simulink model "simulationSprint2"  (R2018b)
settings: Solver=FixedStepAuto  StartTime=0.0  StopTime=10  FixedStep=0.01  MaxStep=100e-3  RelTol=1e-3
(part 1 of 3)
settings Model: Creator=ADEMATO1  LastModifiedBy=afonso
settings SolverCC: PositivePriorityOrder=on  AutoInsertRateTranBlk=on  InsertRTBMode=Always
settings DataIOCC: ReturnWorkspaceOutputs=on
settings DebuggingCC: StringTruncationChecking=warning

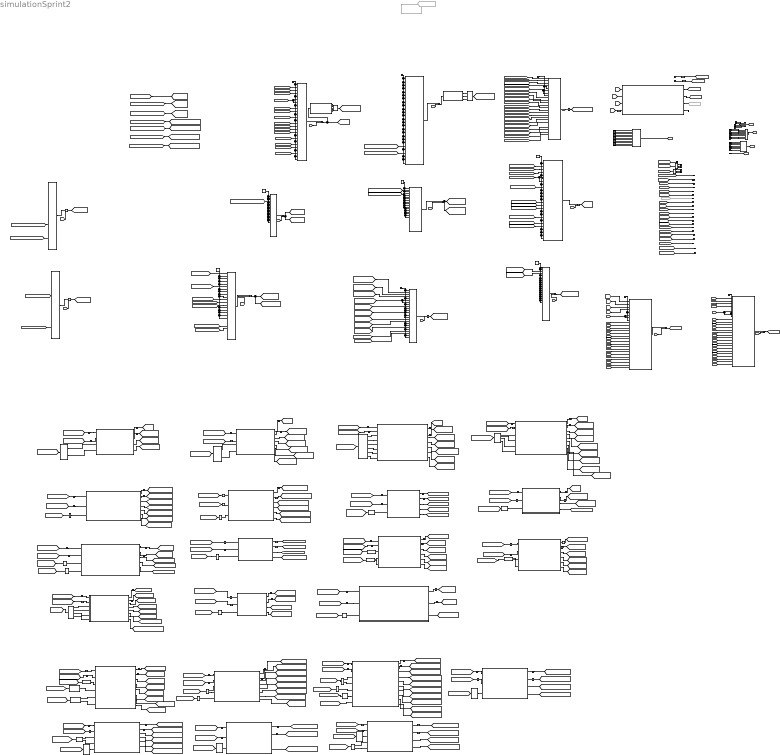
== system simulationSprint2 ==
  note: Test modules .
  note: Multiplexers responsible for redirect of the signal
      | from test modules to select module
  note: Signals Output to the system modules
  note: Signals input from the system modules
  note: This area contains the Select Module and the constants responsible
      | for getting the test number and the begging signal from .m file.
  note: This area contains the multiplexers
      | responsible for redirect the output signals
      | from of test is running.
  note: Mux to output signals
  note: Modules Test
  note: Requeriments Sprint 1 .
  OverHeadLampIn : Inport  OutDataTypeStr=int8
  RearLampIn : Inport  Port=2  OutDataTypeStr=int8
  SyncStatusIn : Inport  Port=3  OutDataTypeStr=int8
  IPCIndicatorIn : Inport  Port=4  OutDataTypeStr=int8
  AjarDoorIndicatorIn : Inport  Port=5  OutDataTypeStr=int8
  SpeedometerIn : Inport  Port=6  OutDataTypeStr=uint8
  OdoMeterIn : Inport  Port=7  OutDataTypeStr=uint8
  GearStateIn : Inport  Port=8  OutDataTypeStr=int8
  HeadLampPark : Inport  Port=9  OutDataTypeStr=int8
  TurnLampsIn : Inport  Port=10  OutDataTypeStr=int8
  DRLampIn : Inport  Port=11  OutDataTypeStr=int8
  MotorStatusIn : Inport  Port=12  OutDataTypeStr=int8
  WindowsFrontLeftIn : Inport  Port=13  OutDataTypeStr=int8
  WindowsFrontRightIn : Inport  Port=14  OutDataTypeStr=int8
  WindowsBackLeftIn : Inport  Port=15  OutDataTypeStr=int8
  WindowsBackRightIn : Inport  Port=16  OutDataTypeStr=int8
  LockFrontLeftIn : Inport  Port=17  OutDataTypeStr=int8
  LockFrontRightIn : Inport  Port=18  OutDataTypeStr=int8
  LockBackLeftIn : Inport  Port=19  OutDataTypeStr=int8
  LockBackRightIn : Inport  Port=20  OutDataTypeStr=int8
  MirrorRightIn : Inport  Port=21  OutDataTypeStr=int8
  MirrorLeftIn : Inport  Port=22  OutDataTypeStr=int8
  HeadLampLowBeamIn : Inport  Port=23  OutDataTypeStr=int8
  HeadLampHighIn : Inport  Port=24  OutDataTypeStr=int8
  TestNumber : Inport  Port=25  OutDataTypeStr=double
  RunTest : Inport  Port=26  OutDataTypeStr=double
  CarLockStateIn : Inport  Port=27  OutDataTypeStr=int8
  BatteryInput : Inport  Port=28  OutDataTypeStr=int8
  trunkIn : Inport  Port=29  OutDataTypeStr=int8
  hoodIn : Inport  Port=30  OutDataTypeStr=int8
  BatterySocIn : Inport  Port=31  OutDataTypeStr=int8
  DistanceToemptyIn : Inport  Port=32  OutDataTypeStr=int8
  GasolineQtyIn : Inport  Port=33  OutDataTypeStr=int8
  KeyCodeIn : Inport  Port=34  OutDataTypeStr=int8
  "\"Req 1\"" : Stateflow chart  TreatAsAtomicUnit=on
  "\"Req 2\"" : Stateflow chart  TreatAsAtomicUnit=on
  Bus Creator : BusCreator  Inputs=11
  Bus Creator1 : BusCreator  Inputs=5
  Bus Creator2 : BusCreator  Inputs=8
  Bus Creator3 : BusCreator  Inputs=7
  Bus Creator4 : BusCreator  Inputs=3
  Bus Creator5 : BusCreator  Inputs=3
  Bus Selector1 : BusSelector  OutputSignals=MotorStatus
  Bus Selector10 : BusSelector  OutputSignals=OverHeadLamp
  Bus Selector11 : BusSelector  OutputSignals=o_s1,o_s2,o_s3
  Bus Selector12 : BusSelector  OutputSignals=LockFrontLeft,LockFrontRight
  Bus Selector13 : BusSelector  OutputSignals=MotorStatus
  Bus Selector14 : BusSelector  OutputSignals=Speedometer
  Bus Selector15 : BusSelector  OutputSignals=RearLamp
  Bus Selector17 : BusSelector  OutputSignals=IPCIndicator
  Bus Selector19 : BusSelector  OutputSignals=AjarDoorIndicator
  Bus Selector2 : BusSelector  OutputSignals=SyncStatus
  Bus Selector21 : BusSelector  OutputSignals=DRLamp,MotorStatus
  Bus Selector22 : BusSelector  OutputSignals=MotorStatus,GearState
  Bus Selector23 : BusSelector  OutputSignals=MotorStatus,HeadLampPark,HeadLampLowBeam,HeadLampHigh
  Bus Selector24 : BusSelector  OutputSignals=MotorStatus,HeadLampPark
  Bus Selector25 : BusSelector  OutputSignals=TurnLamps
  Bus Selector26 : BusSelector  OutputSignals=KeyValue1,KeyValue2,KeyValue3
  Bus Selector27 : BusSelector  OutputSignals=OverHeadLamp
  Bus Selector28 : BusSelector  OutputSignals=RearLamp
  Bus Selector{7,29..30,32,36} (5 alike) : BusSelector  OutputSignals=CarLockState
  Bus Selector3 : BusSelector  OutputSignals=WindowsFrontRight,WindowsFrontLeft
  Bus Selector31 : BusSelector  OutputSignals=hood,trunk
  Bus Selector33 : BusSelector  OutputSignals=BatterySoc
  Bus Selector34 : BusSelector  OutputSignals=DistanceToempty,GasolineQty
  Bus Selector35 : BusSelector  OutputSignals=KeyCodeIn
  Bus Selector4 : BusSelector  OutputSignals=WindowsFrontRight,WindowsFrontLeft
  Bus Selector5 : BusSelector  OutputSignals=MotorStatus
  Bus Selector6 : BusSelector  OutputSignals=LockFrontRight,LockFrontLeft,WindowsFrontLeft,WindowsFrontRight
  Bus Selector8 : BusSelector  OutputSignals=MirrorLeft,MirrorRight,LockBackLeft,LockBackRight,WindowsBackLeft,WindowsBackRight
  Bus Selector9 : BusSelector  OutputSignals=OdoMeter,Speedometer
  Chart : Stateflow chart  TreatAsAtomicUnit=on
  Chart1 : Stateflow chart  Commented=on  TreatAsAtomicUnit=on
  Chart2 : Stateflow chart  TreatAsAtomicUnit=on
  Constant1 : Constant  Value=0  OutDataTypeStr=double
  Constant{2..4,7..8,10} (6 alike) : Constant  Value=0  OutDataTypeStr=int8
  Constant12 : Constant  Value=60  OutDataTypeStr=int8
  Constant5 : Constant  Value=-1  OutDataTypeStr=int8
  Constant6 : Constant  OutDataTypeStr=int8
  Constant9 : Constant  Value=6  OutDataTypeStr=double
  Data Type Conversion : DataTypeConversion
  Data Type Conversion1 : DataTypeConversion  OutDataTypeStr=int8  RndMeth=Ceiling
  Data Type Conversion2 : DataTypeConversion  OutDataTypeStr=int8
  From10 : From  Commented=on  GotoTag=IPCIndicator
  Goto75 : Goto  Commented=on  GotoTag=DDSCommandAux
  Goto8 : Goto  Commented=on  GotoTag=TestResult
  Memory{,1..63,68..91} (88 alike) : Memory
  Mux{,1..9,11..13} (13 alike) : Mux  Inputs=26
  Req 4 : Stateflow chart  TreatAsAtomicUnit=on
  Req10 : Stateflow chart  TreatAsAtomicUnit=on
  Req12 : Stateflow chart  TreatAsAtomicUnit=on
  Req13 : Stateflow chart  TreatAsAtomicUnit=on
  Req14 : Stateflow chart  TreatAsAtomicUnit=on
  Req15 : Stateflow chart  TreatAsAtomicUnit=on
  Req16 : Stateflow chart  TreatAsAtomicUnit=on
  Req17 : Stateflow chart  TreatAsAtomicUnit=on
  Req18 : Stateflow chart  TreatAsAtomicUnit=on
  Req19 : Stateflow chart  TreatAsAtomicUnit=on
  Req21 : Stateflow chart  TreatAsAtomicUnit=on
  Req22 : Stateflow chart  TreatAsAtomicUnit=on
  Req23 : Stateflow chart  TreatAsAtomicUnit=on
  Req24 : Stateflow chart  TreatAsAtomicUnit=on
  Req25 : Stateflow chart  TreatAsAtomicUnit=on
  Req26 : Stateflow chart  TreatAsAtomicUnit=on
  Req3 : Stateflow chart  TreatAsAtomicUnit=on
  Req6 and Req 7 : Stateflow chart  TreatAsAtomicUnit=on
  Req9 : Stateflow chart  TreatAsAtomicUnit=on
  SelectTest : Stateflow chart  TreatAsAtomicUnit=on
  Selector : Selector  InputPortWidth=18  IndexOptions=Index vector (port)  Indices=[1 18]  OutputSizes=1
  Selector{1..9,11..13} (12 alike) : Selector  InputPortWidth=18  IndexOptions=Index vector (port)  Indices=[1 3]  OutputSizes=1
  "SyncWelcomeFeature \"Req 11\"" : Stateflow chart  TreatAsAtomicUnit=on
  Terminator : Terminator
  Terminator1 : Terminator
  KeyfobS1Out : Outport  VectorParamsAs1DForOutWhenUnconnected=on
  KeyfobS2Out : Outport  Port=2  VectorParamsAs1DForOutWhenUnconnected=on
  KeyfobS3Out : Outport  Port=3  VectorParamsAs1DForOutWhenUnconnected=on
  KeyFobCommandsOut : Outport  Port=4  VectorParamsAs1DForOutWhenUnconnected=on
  StartButtomOut : Outport  Port=5  VectorParamsAs1DForOutWhenUnconnected=on
  DoorBackOut : Outport  Port=6  OutDataTypeStr=int8  VectorParamsAs1DForOutWhenUnconnected=on
  DDSCommandOut : Outport  Port=7  VectorParamsAs1DForOutWhenUnconnected=on
  BrakeOut : Outport  Port=8  VectorParamsAs1DForOutWhenUnconnected=on
  DoorFrontOut : Outport  Port=9  OutDataTypeStr=int8  VectorParamsAs1DForOutWhenUnconnected=on
  IPCIndicatorOut : Outport  Port=10  VectorParamsAs1DForOutWhenUnconnected=on
  DoorAjarOut : Outport  Port=11  VectorParamsAs1DForOutWhenUnconnected=on
  GearOut : Outport  Port=12  VectorParamsAs1DForOutWhenUnconnected=on
  WindowLeftOut : Outport  Port=13  VectorParamsAs1DForOutWhenUnconnected=on
  WindowRightOut : Outport  Port=14  VectorParamsAs1DForOutWhenUnconnected=on
  LockRightOut : Outport  Port=15  VectorParamsAs1DForOutWhenUnconnected=on
  LockLeftOut : Outport  Port=16  VectorParamsAs1DForOutWhenUnconnected=on
  HeadLampOut : Outport  Port=17  VectorParamsAs1DForOutWhenUnconnected=on
  LevelLuminosityOut : Outport  Port=18  VectorParamsAs1DForOutWhenUnconnected=on
  TrunkActionOut : Outport  Port=19  VectorParamsAs1DForOutWhenUnconnected=on
  HoodActionOut : Outport  Port=20  VectorParamsAs1DForOutWhenUnconnected=on
  KeyfobOption1Out : Outport  Port=21  VectorParamsAs1DForOutWhenUnconnected=on
  KeyfobOption2Out : Outport  Port=22  VectorParamsAs1DForOutWhenUnconnected=on
  KeyfobOption3Out : Outport  Port=23  VectorParamsAs1DForOutWhenUnconnected=on
  BatteryLevelOut : Outport  Port=24  VectorParamsAs1DForOutWhenUnconnected=on
  EpbOut : Outport  Port=25  VectorParamsAs1DForOutWhenUnconnected=on
  KeyPadOut : Outport  Port=26  VectorParamsAs1DForOutWhenUnconnected=on
  throttleOut : Outport  Port=27  VectorParamsAs1DForOutWhenUnconnected=on
  wires:
  ? -> ?
  [DoorAjarReq13] -> [DoorAjarOut]
  ? -> ?
  "\"Req 2\""/3(o_keyfob) -> [keyfobReq2]
  "\"Req 2\""/1(o_TestResult) -> Memory6/1
  "\"Req 1\""/2(o_testDone) -> Memory3/1
  [EnableTest] -> Memory1/1
  "\"Req 1\""/1(o_TestResult) -> Memory2/1
  "\"Req 1\""/4(o_keyfobCom) -> [keyfobCommandReq1]
  [EnableTest] -> Memory5/1
  "\"Req 2\""/5(o_startButtom) -> [StartButtomReq2]
  [DDCMPDCMSignals] -> Bus Selector4/1
  [DDCMPDCMSignals] -> Bus Selector3/1
  [ReqTest] -> Memory4/1
  "\"Req 2\""/6(o_WindowValue) -> [WindowValueReq2]
  "\"Req 2\""/4(o_keyfobCommand) -> [keyfobCommandReq2]
  "\"Req 2\""/2(o_testDone) -> Memory7/1
  [EnableTest] -> Memory13/1
  Req 4/2(o_testDone) -> Memory15/1
  Req 4/1(o_TestResult) -> Memory14/1
  [ReqTest] -> Memory12/1
  Bus Selector8/2 -> Req3/4(i_mirrorRight)  "<MirrorRight>"
  Bus Selector8/1 -> Req3/3(i_mirrorLeft)  "<MirrorLeft>"
  Req3/3(o_keyfob) -> [KefobFeat3]
  [DDCMPDCMSignals] -> Bus Selector8/1
  Req3/4(o_ddsCommand) -> [ddsCommandFeat3]
  [EnableTest] -> Memory8/1
  [ReqTest] -> Memory9/1
  Req3/1(o_TestResult) -> Memory10/1
  Req3/5(o_keyfobCommand) -> [KeyFobCommandFeat3]
  Req3/2(o_testDone) -> Memory11/1
  Req 4/3(o_keyfob) -> [KeyfobReq4]
  Req 4/4(o_keyfobCom) -> [KeyfobCommReq4]
  Req 4/5(o_lockDoor) -> [LockDoorReq4]
  Req 4/6(o_windowState) -> [WindowStateReq4]
  [DDCMPDCMSignals] -> Bus Selector6/1
  Req6 and Req 7/2(o_testDone) -> Memory29/1
  [BCMSignals] -> Bus Selector10/1
  Bus Selector10/1 -> Req6 and Req 7/3(i_HeadLamp)  "<OverHeadLamp>"
  Req6 and Req 7/1(o_TestResult) -> Memory28/1
  Req6 and Req 7/3(o_keyCommand) -> [KeyCommandReq6]
  Req6 and Req 7/4(o_keyfob) -> [KeyfobReq6]
  Req6 and Req 7/5(o_startButtom) -> [startButtomReq6]
  Req9/2(o_testDone) -> Memory25/1
  Req9/1(o_TestResult) -> Memory24/1
  [HCMAndPCM] -> Bus Selector13/1
  [EnableTest] -> Memory26/1
  [ReqTest] -> Memory27/1
  Bus Selector13/1 -> Req9/3(i_motorState)  "<MotorStatus>"
  Req9/3(o_gear) -> [GearReq9]
  Req9/4(o_keyfob) -> [KeyfobReq9]
  Req9/5(o_keyfobcommand) -> [KeyfobCommReq9]
  Req9/6(o_startButtom) -> [StartButtomReq9]
  Req6 and Req 7/6(o_gear) -> [GearReq6]
  "\"Req 2\""/7(o_gear) -> [gearReq2]
  Bus Selector15/1 -> Req10/3(i_RearLamps)  "<RearLamp>"
  [BCMSignals] -> Bus Selector15/1
  Req10/1(o_TestResult) -> Memory20/1
  Req10/2(o_testDone) -> Memory21/1
  [EnableTest] -> Memory22/1
  [ReqTest] -> Memory23/1
  Req10/3(o_brake) -> [BrakeReq10]
  Req10/4(o_keyfob) -> [KeyFobReq10]
  Req10/5(o_keyfobcom) -> [KeyFobComReq10]
  [ReqTest] -> Memory31/1
  [EnableTest] -> Memory30/1
  [EnableTest] -> Memory19/1
  [IPCAndSync] -> Bus Selector2/1
  "SyncWelcomeFeature \"Req 11\""/2(o_testDone) -> Memory17/1
  "SyncWelcomeFeature \"Req 11\""/3(o_openTheDoor) -> [OpenTheDoorReq11]
  "SyncWelcomeFeature \"Req 11\""/1(o_TestResult) -> Memory16/1
  [ReqTest] -> Memory18/1
  Bus Selector2/1 -> "SyncWelcomeFeature \"Req 11\""/3(i_Sync)  "<SyncStatus>"
  Req12/4(o_keyfobcom) -> [KeyFobComReq12]
  Req12/2(o_testDone) -> Memory35/1
  [ReqTest] -> Memory33/1
  Bus Selector17/1 -> Req12/3(i_IPCInd)  "<IPCIndicator>"
  Req12/1(o_TestResult) -> Memory34/1
  [EnableTest] -> Memory32/1
  Req12/3(o_keyfob) -> [KeyFob12]
  [IPCAndSync] -> Bus Selector17/1
  [IPCAndSync] -> Bus Selector19/1
  Req13/3(o_doorAjar) -> [OpenTheDoorReq13]
  [EnableTest] -> Memory36/1
  [ReqTest] -> Memory37/1
  Req13/1(o_TestResult) -> Memory38/1
  Req13/2(o_testDone) -> Memory39/1
  Bus Selector19/1 -> Req13/3(i_doorAjar)  "<AjarDoorIndicator>"
  Req13/4(o_keyfobcommand) -> [KeyfobCommandReq13]
  [EnableTest] -> Memory40/1
  Req15/2(o_testDone) -> Memory43/1
  [HCMAndPCM] -> Bus Selector22/1
  Req15/1(o_TestResult) -> Memory42/1
  Req15/5(o_keyfobcom) -> [KeyFobComReq15]
  Req15/6(o_startButtom) -> [StartButtomReq15]
  [ReqTest] -> Memory41/1
  Req15/4(o_keyfob) -> [KeyFobReq15]
  Req15/3(o_gear) -> [GerarReq15]
  [HCMAndPCM] -> Bus Selector23/1
  Req16/1(o_TestResult) -> Memory48/1
  Bus Selector23/1 -> Req16/3(i_motorStatus)  "<MotorStatus>"
  Req16/2(o_testDone) -> Memory49/1
  [ReqTest] -> Memory51/1
  Req16/6(o_headLamp) -> [HeadLampReq16]
  [EnableTest] -> Memory50/1
  Req16/3(o_keyfobCom) -> [KeyFobComReq16]
  Req16/4(o_startButtom) -> [StartButtomRq16]
  Req16/5(o_keyfob) -> [KeyFobReq16]
  [ReqTest] -> Memory53/1
  Req17/1(o_TestResult) -> Memory54/1
  Req17/3(o_ketfob) -> [KeyfobReq17]
  [HCMAndPCM] -> Bus Selector25/1
  Bus Selector25/1 -> Req17/3(i_lamp_value)  "<TurnLamps>"
  Req17/4(o_keyfobcom) -> [KeyfobComReq17]
  [EnableTest] -> Memory52/1
  Req17/2(o_testDone) -> Memory55/1
  [DDCMPDCMSignals] -> Bus Selector7/1
  Req18/2(o_testDone) -> Memory45/1
  [EnableTest] -> Memory46/1
  [ReqTest] -> Memory47/1
  Req18/1(o_TestResult) -> Memory44/1
  Bus Selector7/1 -> Req18/3(i_DRL)  "<CarLockState>"
  Req18/3(o_keyfobcom) -> [KeyfobComReq18]
  [TestFinish] -> SelectTest/3(i_done)
  [TestNumber] -> SelectTest/1(i_req)
  SelectTest/2(o_enable) -> [EnableTest]  "EnableTest"
  SelectTest/1(o_req) -> [ReqTest]
  SelectTest/3(o_testResult) -> Goto8/1  "TestResult"
  Mux/1 -> Selector/1
  [keyfobReq2] -> Mux/2
  [KefobFeat3] -> Mux/3
  [KeyfobReq4] -> Mux/4
  [KeyfobReq6] -> Mux/6, Mux/7
  [KeyfobReq9] -> Mux/9
  [KeyFobReq10] -> Mux/10
  [KeyFobReq15] -> Mux/15
  [KeyFobReq16] -> Mux/16
  [KeyfobReq17] -> Mux/17
  ? -> ?
  [StartButtomReq2] -> Mux1/2
  [StartButtomReq9] -> Mux1/9
  [startButtomReq6] -> Mux1/7, Mux1/6
  [TestNumber] -> Selector1/2
  Mux1/1 -> Selector1/1
  Selector1/1 -> [StartButtomOut]
  Constant3/1 -> Mux1/5, Mux1/11, Mux1/13, Mux1/24, Mux1/23, Mux1/20, Mux1/18, Mux1/17, Mux1/12, Mux1/10, Mux1/8, Mux1/1
  Constant2/1 -> Mux/13, Mux/26, Mux/25, Mux/23, Mux/20, Mux/18, Mux/11, Mux/8, Mux/5, Mux/1
  [StartButtomReq15] -> Mux1/15
  [StartButtomRq16] -> Mux1/16
  [TestNumber] -> Selector3/2
  Mux3/1 -> Selector3/1
  [gearReq2] -> Mux3/2
  [GearReq6] -> Mux3/7, Mux3/6
  [GearReq9] -> Mux3/9
  [GerarReq15] -> Mux3/15
  Selector3/1 -> [GearOut]
  Mux4/1 -> Selector4/1
  [TestNumber] -> Selector4/2
  Selector4/1 -> [WindowRightOut], [WindowLeftOut]
  [WindowValueReq2] -> Mux4/2
  [WindowStateReq4] -> Mux4/4
  Selector7/1 -> [LockRightOut], [LockLeftOut]
  [Req1Done] -> Mux6/1
  Selector6/1 -> [TestFinish]
  Bus Selector22/1 -> Req15/3(i_motorStatus)  "<MotorStatus>"
  RearLampIn/1 -> Bus Creator1/2  "RearLamp"
  OverHeadLampIn/1 -> Bus Creator1/1  "OverHeadLamp"
  Bus Creator1/1 -> [BCMSignals]  "BCMSignals"
  Bus Creator2/1 -> [IPCAndSync]  "IPCAndSync"
  OdoMeterIn/1 -> Bus Creator2/5  "OdoMeter"
  IPCIndicatorIn/1 -> Bus Creator2/2  "IPCIndicator"
  SpeedometerIn/1 -> Bus Creator2/4  "Speedometer"
  AjarDoorIndicatorIn/1 -> Bus Creator2/3  "AjarDoorIndicator"
  SyncStatusIn/1 -> Bus Creator2/1  "SyncStatus"
  TurnLampsIn/1 -> Bus Creator3/3  "TurnLamps"
  DRLampIn/1 -> Bus Creator3/4  "DRLamp"
  GearStateIn/1 -> Bus Creator3/1  "GearState"
  MotorStatusIn/1 -> Bus Creator3/5  "MotorStatus"
  HeadLampPark/1 -> Bus Creator3/2  "HeadLampPark"
  Bus Creator3/1 -> [HCMAndPCM]  "HCMAndPCM"
  LockBackRightIn/1 -> Bus Creator/8  "LockBackRight"
  LockFrontLeftIn/1 -> Bus Creator/5  "LockFrontLeft"
  LockBackLeftIn/1 -> Bus Creator/7  "LockBackLeft"
  MirrorRightIn/1 -> Bus Creator/9  "MirrorRight"
  WindowsBackLeftIn/1 -> Bus Creator/3  "WindowsBackLeft"
  MirrorLeftIn/1 -> Bus Creator/10  "MirrorLeft"
  WindowsFrontLeftIn/1 -> Bus Creator/1  "WindowsFrontLeft"
  WindowsBackRightIn/1 -> Bus Creator/4  "WindowsBackRight"
  Bus Creator/1 -> [DDCMPDCMSignals]  "DDCMPDCMSignals"
  LockFrontRightIn/1 -> Bus Creator/6  "LockFrontRight"
  WindowsFrontRightIn/1 -> Bus Creator/2  "WindowsFrontRight"
  [HeadLampOut] -> HeadLampOut/1  "HeadLampOut"
  From10/1 -> IPCIndicatorOut/1
  [WindowLeftOut] -> WindowLeftOut/1  "WindowLeftOut"
  [GearOut] -> GearOut/1  "GearOut"
  [DDSCommandOut] -> DDSCommandOut/1  "DDSCommandOut"
  [LockRightOut] -> LockRightOut/1  "LockRightOut"
  [DoorFrontOut] -> DoorFrontOut/1  "DoorFrontOut"
  [LockLeftOut] -> LockLeftOut/1  "LockLeftOut"
  [DoorBackOut] -> DoorBackOut/1  "DoorBackOut"
  [BreakOut] -> BrakeOut/1  "BreakOut"
  [WindowRightOut] -> WindowRightOut/1  "WindowRightOut"
  [DoorAjarOut] -> DoorAjarOut/1  "DoorAjarOut"
  [KeyfobCommandsOut] -> KeyFobCommandsOut/1  "KeyfobCommandsOut"
  [StartButtomOut] -> StartButtomOut/1  "StartButtomOut"
  Mux5/1 -> Selector5/1
  [TestNumber] -> Selector5/2
  Selector5/1 -> [ResultTest]
  [Req1Ok] -> Mux5/1
  [Req3Ok] -> Mux5/3
  [Req4Ok] -> Mux5/4
  [Req6Ok] -> Mux5/7, Mux5/6
  [Req9Ok] -> Mux5/9
  [Req10Ok] -> Mux5/10
  [Req11Ok] -> Mux5/11
  [Req12Ok] -> Mux5/12
  [Req13Ok] -> Mux5/13
  [Req15Ok] -> Mux5/15
  [Req17Ok] -> Mux5/17
  [Req18Ok] -> Mux5/18
  [Req16Ok] -> Mux5/16
  Constant7/1 -> Mux5/8, Mux5/5
  [ResultTest] -> Data Type Conversion/1
  Data Type Conversion/1 -> SelectTest/4(i_testResult)
  [Req2Done] -> Mux6/2
  [Req3Done] -> Mux6/3
  [Req4Done] -> Mux6/4
  [Req6Done] -> Mux6/7, Mux6/6
  [Req9Done] -> Mux6/9
  [Req10Done] -> Mux6/10
  [Req11Done] -> Mux6/11
  [Req12Done] -> Mux6/12
  [Req13Done] -> Mux6/13
  [Req15Done] -> Mux6/15
  [Req16Done] -> Mux6/16
  [Req17Done] -> Mux6/17
  [Req18Done] -> Mux6/18
  [TestNumber] -> Selector6/2
  Mux6/1 -> Selector6/1
  Constant8/1 -> Mux6/8, Mux6/5
  Memory/1 -> "\"Req 1\""/1(i_desiredTest)
  [ReqTest] -> Memory/1
  Memory1/1 -> "\"Req 1\""/2(i_enable)
  Memory2/1 -> [Req1Ok]
  Memory3/1 -> [Req1Done]
  Memory4/1 -> "\"Req 2\""/1(i_desiredTest)
  Memory5/1 -> "\"Req 2\""/2(i_enable)
  Memory6/1 -> [Req2Ok]
  Memory7/1 -> [Req2Done]
  Memory8/1 -> Req3/1(i_enable)
  Memory9/1 -> Req3/2(i_desiredTest)
  Memory10/1 -> [Req3Ok]
  Memory11/1 -> [Req3Done]
  Memory12/1 -> Req 4/1(i_desiredTest)
  Memory13/1 -> Req 4/2(i_enable)
  Memory14/1 -> [Req4Ok]
  Memory15/1 -> [Req4Done]
  Memory16/1 -> [Req11Ok]
  Memory17/1 -> [Req11Done]
  Memory18/1 -> "SyncWelcomeFeature \"Req 11\""/1(i_desiredTest)
  Memory19/1 -> "SyncWelcomeFeature \"Req 11\""/2(i_enable)
  Memory20/1 -> [Req10Ok]
  Memory21/1 -> [Req10Done]
  Memory22/1 -> Req10/1(i_enable)
  Memory23/1 -> Req10/2(i_desiredTest)
  Memory24/1 -> [Req9Ok]
  Memory25/1 -> [Req9Done]
  Memory26/1 -> Req9/1(i_enable)
  Memory27/1 -> Req9/2(i_desiredTest)
  Memory28/1 -> [Req6Ok]
  Memory29/1 -> [Req6Done]
  Memory30/1 -> Req6 and Req 7/1(i_enable)
  Memory31/1 -> Req6 and Req 7/2(i_DesiredTest)
  Memory32/1 -> Req12/1(i_enable)
  Memory33/1 -> Req12/2(i_desiredTest)
  Memory34/1 -> [Req12Ok]
  Memory35/1 -> [Req12Done]
  Memory36/1 -> Req13/1(i_enable)
  Memory37/1 -> Req13/2(i_desiredTest)
  Memory38/1 -> [Req13Ok]
  Memory39/1 -> [Req13Done]
  Memory40/1 -> Req15/1(i_enable)
  Memory41/1 -> Req15/2(i_desiredTest)
  Memory42/1 -> [Req15Ok]
  Memory43/1 -> [Req15Done]
  Memory44/1 -> [Req18Ok]
  Memory45/1 -> [Req18Done]
  Memory46/1 -> Req18/1(i_enable)
  Memory47/1 -> Req18/2(i_desiredTest)
  Memory48/1 -> [Req16Ok]
  Memory49/1 -> [Req16Done]
  Memory50/1 -> Req16/1(i_enable)
  Memory51/1 -> Req16/2(i_desiredTest)
  Memory52/1 -> Req17/1(i_enable)
  Memory53/1 -> Req17/2(i_desiredTest)
  Memory54/1 -> [Req17Ok]
  Memory55/1 -> [Req17Done]
  Memory57/1 -> Req14/2(i_desiredTest)
  Memory59/1 -> [Req14Done]
  Req14/4(o_keyfob) -> [KeyFobReq14]
  Memory58/1 -> [Req14Ok]
  Memory56/1 -> Req14/1(i_enable)
  Req14/3(o_gear) -> [GerarReq14]
  Bus Selector1/1 -> Req14/3(i_motorStatus)  "<MotorStatus>"
  [EnableTest] -> Memory56/1
  [ReqTest] -> Memory57/1
  Req14/1(o_TestResult) -> Memory58/1
  Req14/5(o_keyfobcom) -> [KeyFobComReq14]
  [HCMAndPCM] -> Bus Selector1/1
  Req14/6(o_startButtom) -> [StartButtomReq14]
  Req14/2(o_testDone) -> Memory59/1
  [IPCAndSync] -> Bus Selector9/1
  Bus Selector9/1 -> Req14/4(i_odometer)  "<OdoMeter>"
  Bus Selector9/2 -> Req14/5(i_speedmeter)  "<Speedometer>"
  [KeyFob12] -> Mux/12
  [KeyFobReq14] -> Mux/14
  [StartButtomReq14] -> Mux1/14
  [GerarReq14] -> Mux3/14
  [Req14Ok] -> Mux5/14
  [Req14Done] -> Mux6/14
  [RunTest] -> SelectTest/2(i_enable)
  TestNumber/1 -> Data Type Conversion1/1
  RunTest/1 -> Data Type Conversion2/1
  SelectTest/4(o_testEnd) -> Terminator1/1  "TestEnd"
  [Req2Ok] -> Mux5/2
  "SyncWelcomeFeature \"Req 11\""/4(o_KeyfobCommand) -> [KeyFobComReq11]
  Chart/1(o_s1) -> Bus Creator4/1  "o_s1"
  Chart/2(o_s2) -> Bus Creator4/2  "o_s2"
  Chart/3(o_s3) -> Bus Creator4/3  "o_s3"
  Selector/1 -> Chart/1(i_keyfobValue), [KeyfobOut]
  Bus Creator4/1 -> [KeyfobOutToModule]
  [KeyfobOut] -> Terminator/1  "KeyfobOut"
  Bus Selector22/2 -> Req15/4(i_gear)  "<GearState>"
  Bus Selector23/2 -> Req16/4(i_headLampPark)  "<HeadLampPark>"
  Req16/7(o_levelluminosity) -> [levelLuminosityReq16]
  [levelLuminosityReq16] -> LevelLuminosityOut/1  "levelLuminosityOut"
  HeadLampLowBeamIn/1 -> Bus Creator3/6  "HeadLampLowBeam"
  HeadLampHighIn/1 -> Bus Creator3/7  "HeadLampHigh"
  Bus Selector23/4 -> Req16/6(i_headLampHigh)  "<HeadLampHigh>"
  Bus Selector23/3 -> Req16/5(i_headLampLowBeam)  "<HeadLampLowBeam>"
  [KeyfobOutToModule] -> Bus Selector11/1
  Bus Selector11/1 -> KeyfobS1Out/1  "<o_s1>"
  Bus Selector11/2 -> KeyfobS2Out/1  "<o_s2>"
  Bus Selector11/3 -> KeyfobS3Out/1  "<o_s3>"
  [startButtomReq4] -> Mux1/4
  Req 4/7(o_startButtom) -> [startButtomReq4]
  Data Type Conversion2/1 -> [RunTest]
  [TestNumber] -> Selector/2  "here"
  Data Type Conversion1/1 -> [TestNumber]
  [LockDoorReq4] -> Mux7/4
  "\"Req 1\""/3(o_CloseDoor) -> [OpenTheDoorReq1]
  [TestNumber] -> Selector7/2
  Mux7/1 -> Selector7/1
  Bus Selector3/2 -> "\"Req 1\""/4(i_WindowLeftState)  "<WindowsFrontLeft>"
  Bus Selector3/1 -> "\"Req 1\""/3(i_WindowRightState)  "<WindowsFrontRight>"
  Bus Selector4/1 -> "\"Req 2\""/3(i_WindowRightState)  "<WindowsFrontRight>"
  Bus Selector4/2 -> "\"Req 2\""/4(i_WindowLeftState)  "<WindowsFrontLeft>"
  Bus Selector6/1 -> Req 4/3(i_stateDoorRight)  "<LockFrontRight>"
  Bus Selector6/2 -> Req 4/4(i_stateDoorLeft)  "<LockFrontLeft>"
  Bus Selector6/3 -> Req 4/5(i_windowStateLeft)  "<WindowsFrontLeft>"
  Bus Selector6/4 -> Req 4/6(i_windowStateRight)  "<WindowsFrontRight>"
  Req 4/8(o_DDSCommand) -> [ddsCommandReq4]
  [ddsCommandReq4] -> Mux8/4
  [ddsCommandFeat3] -> Mux8/3
  [TestNumber] -> Selector8/2
  Mux8/1 -> Selector8/1
  Selector8/1 -> [DDSCommandOut]
  Req 4/9(o_gear) -> [GearReq4]
  [GearReq4] -> Mux3/4
  Req3/6(o_startButtom) -> [startButtomReq3]
  Req3/7(o_gear) -> [GearReq3]
  [GearReq3] -> Mux3/3
  [startButtomReq3] -> Mux1/3
  [OpenTheDoorReq11] -> Mux9/11
  [OpenTheDoorReq6] -> Mux9/6
  [TestNumber] -> Selector9/2
  Mux9/1 -> Selector9/1
  Selector9/1 -> [DoorBackOut], [DoorFrontOut]
  Req6 and Req 7/7(o_door) -> [OpenTheDoorReq6]
  [OpenTheDoorReq13] -> Mux9/13
  Req16/8(o_gear) -> [GerarReq16]
  [GerarReq16] -> Mux3/16
  [OpenTheDoorReq1] -> Mux9/1
  Req12/5(o_doorCom) -> [OpenTheDoorReq12]
  [OpenTheDoorReq12] -> Mux9/12
  Req19/1(o_TestResult) -> Memory62/1
  [EnableTest] -> Memory60/1
  Memory61/1 -> Req19/2(i_desiredTest)
  [DDCMPDCMSignals] -> Bus Selector12/1
  [ReqTest] -> Memory61/1
  Req19/5(o_keyfobcom) -> [KeyFobComReq19]
  Memory63/1 -> [Req19Done]
  Req19/6(o_startButtom) -> [StartButtomReq19]
  Bus Selector5/1 -> Req19/3(i_motorStatus)  "<MotorStatus>"
  Req19/4(o_keyfob) -> [KeyFobReq19]
  [HCMAndPCM] -> Bus Selector5/1
  Req19/3(o_gear) -> [GerarReq19]
  Memory60/1 -> Req19/1(i_enable)
  Memory62/1 -> [Req19Ok]
  Req19/2(o_testDone) -> Memory63/1
  [IPCAndSync] -> Bus Selector14/1
  Bus Selector14/1 -> Req19/4(i_speed)  "<Speedometer>"
  Bus Selector12/1 -> Req19/5(i_LeftBackDoorLockState)  "<LockFrontLeft>"
  Bus Selector12/2 -> Req19/6(i_RightBackDoorLockState)  "<LockFrontRight>"
  Req19/7(o_throttle) -> [throttleReq19]
  Mux11/1 -> Selector11/1
  [TestNumber] -> Selector11/2
  Constant12/1 -> Mux11/1, Mux11/2, Mux11/3, Mux11/4, Mux11/6, Mux11/7, Mux11/9, Mux11/10, Mux11/11, Mux11/26, Mux11/25, Mux11/24, Mux11/22, Mux11/20, Mux11/19, Mux11/18, Mux11/17, Mux11/16, Mux11/15, Mux11/14, Mux11/13, Mux11/12, Mux11/8, Mux11/5
  Bus Selector8/3 -> Req3/5(i_LeftDoorBackLockState)  "<LockBackLeft>"
  Bus Selector8/4 -> Req3/6(i_RightDoorBackLockState)  "<LockBackRight>"
  Bus Selector8/5 -> Req3/7(i_LeftWindowBackState)  "<WindowsBackLeft>"
  Bus Selector8/6 -> Req3/8(i_RightWindowBackState)  "<WindowsBackRight>"
  Req21/1(o_TestResult) -> Memory68/1
  Req21/2(o_testDone) -> Memory69/1
  Req21/6(o_startButtom) -> [StartButtomReq21]
  [EnableTest] -> Memory70/1
  Memory68/1 -> [Req21Ok]
  Req21/4(o_keyfob) -> [KeyfobReq21]
  Req21/5(o_keyfobcommand) -> [KeyfobCommReq21]
  Req21/3(o_gear) -> [GearReq21]
  [ReqTest] -> Memory71/1
  Memory71/1 -> Req21/2(i_desiredTest)
  Bus Selector21/1 -> Req21/3(i_CarLockState)  "<DRLamp>"
  [HCMAndPCM] -> Bus Selector21/1
  Memory69/1 -> [Req21Done]
  Memory70/1 -> Req21/1(i_enable)
  CarLockStateIn/1 -> Bus Creator/11  "CarLockState"
  Bus Selector21/2 -> Req21/4(i_MotorStatus)  "<MotorStatus>"
  Req22/5(o_keyfobcommand) -> [KeyfobCommReq22]
  [HCMAndPCM] -> Bus Selector24/1
  Memory72/1 -> [Req22Ok]
  Req22/1(o_TestResult) -> Memory72/1
  Memory74/1 -> Req22/1(i_enable)
  Req22/6(o_startButtom) -> [StartButtomReq22]
  Memory73/1 -> [Req22Done]
  Req22/4(o_keyfob) -> [KeyfobReq22]
  Memory75/1 -> Req22/2(i_desiredTest)
  Req22/3(o_gear) -> [GearReq22]
  Req22/2(o_testDone) -> Memory73/1
  [EnableTest] -> Memory74/1
  Bus Selector24/1 -> Req22/3(i_motorState)  "<MotorStatus>"
  [ReqTest] -> Memory75/1
  Memory76/1 -> [Req23Ok]
  Req23/2(o_testDone) -> Memory77/1
  Memory78/1 -> Req23/1(i_enable)
  Req23/3(o_keyfobcommand) -> [KeyfobCommReq23]
  Memory79/1 -> Req23/2(i_desiredTest)
  [ReqTest] -> Memory79/1
  [EnableTest] -> Memory78/1
  Memory77/1 -> [Req23Done]
  Req23/1(o_TestResult) -> Memory76/1
  [ReqTest] -> Memory83/1
  Req24/3(o_keyfobcommand) -> [KeyfobCommReq24]
  Memory80/1 -> [Req24Ok]
  Req24/2(o_testDone) -> Memory81/1
  Memory82/1 -> Req24/1(i_enable)
  Memory83/1 -> Req24/2(i_desiredTest)
  Memory81/1 -> [Req24Done]
  [EnableTest] -> Memory82/1
  Req24/1(o_TestResult) -> Memory80/1
  Req25/1(o_TestResult) -> Memory84/1
  Memory84/1 -> [Req25Ok]
  Req25/2(o_testDone) -> Memory85/1
  Memory87/1 -> Req25/2(i_desiredTest)
  Memory86/1 -> Req25/1(i_enable)
  [ReqTest] -> Memory87/1
  Memory85/1 -> [Req25Done]
  [EnableTest] -> Memory86/1
  Req23/4(o_keyfobCode) -> [KeyfobCodeReq23]
  Req24/4(o_keyfobCode) -> [KeyfobReq24]
  Req24/5(o_trunkState) -> [TrunkAction24]
  Req24/6(o_hoodState) -> [HoodAction24]
  Req25/3(o_keyfobCode) -> [KeyPadReq25]
  Req21/8(o_doorAction) -> [OpenTheDoorReq21]
  Req21/7(o_keyfobCode) -> [KeyfobCodeReq21]
  Req22/7(o_DoorAction) -> [OpenTheDoorReq22]
  Memory91/1 -> Req26/2(i_desiredTest)
  [EnableTest] -> Memory90/1
  Req26/1(o_TestResult) -> Memory88/1
  [ReqTest] -> Memory91/1
  Memory88/1 -> [Req26Ok]
  Req26/2(o_testDone) -> Memory89/1
  Memory89/1 -> [Req26Done]
  Memory90/1 -> Req26/1(i_enable)
  [Req19Ok] -> Mux5/19
  [Req20Ok] -> Mux5/20
  [Req22Ok] -> Mux5/22
  [Req21Ok] -> Mux5/21
  [Req23Ok] -> Mux5/23
  [Req24Ok] -> Mux5/24
  [Req25Ok] -> Mux5/25
  [Req26Ok] -> Mux5/26
  [Req19Done] -> Mux6/19
  [Req20Done] -> Mux6/20
  [Req21Done] -> Mux6/21
  [Req22Done] -> Mux6/22
  [Req23Done] -> Mux6/23
  [Req24Done] -> Mux6/24
  [Req25Done] -> Mux6/25
  [Req26Done] -> Mux6/26
  [KeyFobComReq11] -> Mux2/11
  [KeyFobComReq16] -> Mux2/16
  Selector2/1 -> [KeyfobCommandsOut]
  [KeyfobCommReq4] -> Mux2/4
  [KeyfobComReq17] -> Mux2/17
  [keyfobCommandReq2] -> Mux2/2
  [TestNumber] -> Selector2/2
  [KeyfobCommandReq13] -> Mux2/13
  [keyfobCommandReq1] -> Mux2/1
  [KeyfobCommReq9] -> Mux2/9
  [KeyfobComReq18] -> Mux2/18
  Constant6/1 -> Mux2/8, Mux2/5
  Mux2/1 -> Selector2/1
  [KeyCommandReq6] -> Mux2/7, Mux2/6
  [KeyFobCommandFeat3] -> Mux2/3
  [KeyFobComReq14] -> Mux2/14
  [KeyFobComReq15] -> Mux2/15
  [KeyFobComReq10] -> Mux2/10
  [KeyFobComReq12] -> Mux2/12
  Constant4/1 -> Mux3/24, Mux3/25, Mux3/26, Mux3/23, Mux3/20, Mux3/18, Mux3/17, Mux3/13, Mux3/12, Mux3/11, Mux3/10, Mux3/8, Mux3/5, Mux3/1
  [GerarReq19] -> Mux3/19
  [KeyFobComReq19] -> Mux2/19
  [KeyFobReq19] -> Mux/19
  Constant5/1 -> Mux4/5, Mux4/7, Mux4/18, Mux4/17, Mux4/16, Mux4/15, Mux4/14, Mux4/13, Mux4/12, Mux4/11, Mux4/10, Mux4/9, Mux4/8, Mux4/6, Mux4/3, Mux4/1
  Constant9/1 -> Mux8/1, Mux8/5, Mux8/6, Mux8/7, Mux8/8, Mux8/9, Mux8/10, Mux8/11, Mux8/12, Mux8/13, Mux8/14, Mux8/15, Mux8/16, Mux8/17, Mux8/18, Mux8/2
  [StartButtomReq19] -> Mux1/19
  Constant1/1 -> Mux7/1, Mux7/2, Mux7/3, Mux7/5, Mux7/6, Mux7/7, Mux7/8, Mux7/9, Mux7/10, Mux7/11, Mux7/12, Mux7/13, Mux7/14, Mux7/15, Mux7/16, Mux7/17, Mux7/18
  Constant10/1 -> Mux9/2, Mux9/3, Mux9/4, Mux9/5, Mux9/7, Mux9/8, Mux9/9, Mux9/10, Mux9/15, Mux9/16, Mux9/17, Mux9/18, Mux9/14
  [TrunkAction24] -> [TrunkActionOut]
  [HoodAction24] -> [HoodActionOut]
  [TrunkActionOut] -> TrunkActionOut/1  "TrunkActionOut"
  [HoodActionOut] -> HoodActionOut/1  "HoodActionOut"
  [KeyfobReq21] -> Mux/21
  [KeyfobReq22] -> Mux/22
  [KeyfobReq24] -> Mux/24
  [OpenTheDoorReq21] -> Mux9/21
  [StartButtomReq21] -> Mux1/21
  [StartButtomReq22] -> Mux1/22
  [KeyfobCommReq21] -> Mux2/21
  [KeyfobCommReq22] -> Mux2/22
  [KeyfobCommReq23] -> Mux2/23
  [KeyfobCommReq24] -> Mux2/24
  [GearReq21] -> Mux3/21
  [GearReq22] -> Mux3/22
  [KeyfobCodeReq21] -> Mux11/21
  [KeyfobCodeReq23] -> Mux11/23
  Selector11/1 -> Chart2/1(i_codeKey)  "KeyfobCode"
  Chart2/1(o_keyValue1) -> Bus Creator5/1  "KeyValue1"
  Chart2/2(o_keyValue2) -> Bus Creator5/2  "KeyValue2"
  Chart2/3(o_keyValue3) -> Bus Creator5/3  "KeyValue3"
  Bus Creator5/1 -> [KeyfobOption]
  [KeyfobOption] -> Bus Selector26/1
  Bus Selector26/1 -> KeyfobOption1Out/1  "<KeyValue1>"
  Bus Selector26/2 -> KeyfobOption2Out/1  "<KeyValue2>"
  Bus Selector26/3 -> KeyfobOption3Out/1  "<KeyValue3>"
  [BCMSignals] -> Bus Selector27/1
  Bus Selector27/1 -> Req22/5(i_OverHeadLamp)  "<OverHeadLamp>"
  Bus Selector24/2 -> Req22/4(i_headLampPark)  "<HeadLampPark>"
  [BCMSignals] -> Bus Selector28/1
  Bus Selector28/1 -> Req22/6(i_RearLamp)  "<RearLamp>"
  BatteryInput/1 -> [BatteryLevel]  "BatteryLevel"
  [BatteryLevel] -> Req22/7(i_battery)
  Req22/8(o_battery) -> [batteryLevelReq22]
  Req22/10(o_brake) -> [BrakeReq22]
  Req22/9(o_HeadLamp) -> [HeadLampReq22]
  [OpenTheDoorReq22] -> Mux9/22
  Mux12/1 -> Selector12/1
  Selector12/1 -> [BreakOut]
  [TestNumber] -> Selector12/2
  [BrakeReq10] -> Mux12/10
  [BrakeReq22] -> Mux12/22
  Selector13/1 -> [HeadLampOut]
  Mux13/1 -> Selector13/1
  [TestNumber] -> Selector13/2
  [HeadLampReq16] -> Mux13/17
  [HeadLampReq22] -> Mux13/22
  [batteryLevelReq22] -> [batteryLevel]
  [batteryLevel] -> BatteryLevelOut/1  "BatteryLevelOut"
  [DDCMPDCMSignals] -> Bus Selector29/1
  Bus Selector29/1 -> Req23/3(i_CarLockStatus)  "<CarLockState>"
  Bus Selector30/1 -> Req24/5(i_CarLockStatus)  "<CarLockState>"
  [DDCMPDCMSignals] -> Bus Selector30/1
  trunkIn/1 -> Bus Creator1/3  "trunk"
  hoodIn/1 -> Bus Creator1/4  "hood"
  [BCMSignals] -> Bus Selector31/1
  Bus Selector31/2 -> Req24/4(i_trunkState)  "<trunk>"
  Bus Selector31/1 -> Req24/3(i_hoodState)  "<hood>"
  BatterySocIn/1 -> Bus Creator2/6  "BatterySoc"
  [IPCAndSync] -> Bus Selector33/1
  Req26/3(o_keyfobcommand) -> [KeyfobReq26]
  Req26/4(o_keyfobCode) -> [KeyfobCommReq26]
  Bus Selector33/1 -> Req12/4(i_batterySocWarning)  "<BatterySoc>"
  DistanceToemptyIn/1 -> Bus Creator2/7  "DistanceToempty"
  Bus Selector34/1 -> Req26/4(i_distance)  "<DistanceToempty>"
  [IPCAndSync] -> Bus Selector34/1
  Bus Selector32/1 -> Req26/3(i_CarLockStatus)  "<CarLockState>"
  [DDCMPDCMSignals] -> Bus Selector32/1
  GasolineQtyIn/1 -> Bus Creator2/8  "GasolineQty"
  Bus Selector34/2 -> Req26/5(i_gasolineQty)  "<GasolineQty>"
  KeyCodeIn/1 -> Bus Creator1/5  "KeyCodeIn"
  Bus Selector35/1 -> Req21/5(i_pcmKeyCodeTest)  "<KeyCodeIn>"
  [BCMSignals] -> Bus Selector35/1
  Req19/8(o_epb) -> [epbReq19]
  [epbReq19] -> [epb]
  [epb] -> EpbOut/1  "Epb"
  Bus Selector36/1 -> Req25/3(i_CarLockStatus)  "<CarLockState>"
  [DDCMPDCMSignals] -> Bus Selector36/1
  [KeyPadReq25] -> [KeyPad]
  [KeyPad] -> KeyPadOut/1  "KeyPad"
  [throttleReq19] -> [throttle]
  [throttle] -> throttleOut/1  "throttle"

== stateflow chart simulationSprint2/Req14 ==
  note: The module responsible by test the requeriment fourteen.
      |
      | Notice : i_ means input signals
      | 		o_ means output signals
      |
      | Input :
      | i_enable - Start the test. 1- Start test . 0 - Do nothing.
      | i_desiredTest - Test Number Value. All the modules recieve the
      | signal and decide either execute the test. Ex: Value "1" means that will being testing the requeriment 1.
      | i_MotorState. 1 - On ; 0 - Off .
      | i_speedmeter - Showing speed of the car . Range - 0 ~ 220 km/h
      | i_odometer - Showing odometer of the car . Range - 0 ~ 10 Km.
      |
      | Output :
      | o_TestResult - Result of test. 1 - Test ran correctly ; 0 - Test ran incorrectly.
      | o_TestDone - Test has been completed. 1 - Completed ;
      | o_keyfobComm - Signal to lock or unlock the car. "1 - lock the car ; 2 - Unlock the car" ;  0 - Do nothing.
      | o_startButtom - Signal to start or off the car. 1- Car Start ; 0 - Car off.
      | o_keyfob - Signal that indicates if the key is inside or not from the car. 1 - Key inside ; 0 - Key outside.
      | o_gear = gear State ; 1 - Park ; 0 - Engaged.
  state state_gearParkOnCar
    entry:r_aux=0;
    during:
    o_keyfobcom = 2;
    on after(50,msec):
    o_keyfobcom = 0;
    on after(200,msec):
    o_keyfob =1;
    o_gear=1;
    on after(300,msec):
    o_startButtom =1;
    on after(1,sec):
    r_aux=1;
    exit :
    r_speedmeter = i_speedmeter ;
    r_odometer = i_odometer;
    r_aux=0;
  state state_idle
    entry:
    r_aux=0;
  state state_testSpeedmeter
    entry :
    r_error = 0;
    during :
    if (i_speedmeter<r_speedmeter || i_odometer < r_odometer || (i_odometer > r_odometer+20) || (i_speedmeter>r_speedmeter+20))
    r_error = 1;
    end
    if (i_speedmeter >220)
    r_error = 1 ;
    r_aux = 0 ;
    else if (i_speedmeter == 220)
    r_aux =1 ;
    end
    end
    r_speedmeter = i_speedmeter ;
    r_odometer=i_odometer;
    exit :
    r_aux = 0 ;
    r_error = 0 ;
  state State_error
    during:
    o_TestResult =0;
    o_testDone =1 ;
    on after(300,msec):
    r_aux =1;
    exit :
    r_aux =0;
  state state_testSpeedmeter1
    entry :
    r_error = 0;
    during :
    if (i_speedmeter>r_speedmeter || i_odometer > r_odometer || (i_speedmeter< r_speedmeter -20) || (i_odometer < r_odometer - 20))
    r_error = 1;
    end
    if (i_speedmeter < 0 )
    r_error = 1 ;
    r_aux =0 ;
    else if (i_speedmeter == 0)
    r_aux =1 ;
    end
    end
    r_speedmeter = i_speedmeter ;
    r_odometer =i_odometer;
    exit :
    r_aux = 0 ;
    r_error = 0
  state State_feat_ok
    during:
    o_TestResult =1;
    o_testDone =1;
    on after(100,msec):
    r_aux =1;
    exit:
    r_aux =0;
  state state_update
    entry:
    r_aux = 0;
    on after(200,msec):
    during:
    o_TestResult =0;
    o_testDone = 0;
    r_aux =1 ;
    exit:
    o_keyfob = 0 ;
    o_keyfobcom = 0;
    o_gear = 0 ;
    o_startButtom = 0 ;
  (default) -> state_idle
  state_idle -> state_gearParkOnCar : [i_enable==1 && i_desiredTest == 14]
  state_update -> state_idle : [r_aux==1]
  state_gearParkOnCar -> State_error [order 2] : [r_aux==1 && i_motorStatus==0]
  state_gearParkOnCar -> state_testSpeedmeter [order 1] : [r_aux==1 && i_motorStatus==1]
  state_testSpeedmeter -> State_error [order 2] : [after(1.5,sec) && r_error ==1]
  State_error -> state_update : [r_aux==1]
  state_testSpeedmeter1 -> State_error [order 1] : [after(1.5,sec) && r_error ==1]
  state_testSpeedmeter -> state_testSpeedmeter1 [order 1] : [after(1.5,sec) && r_aux==1 && r_error ==0]
  state_testSpeedmeter1 -> State_feat_ok [order 2] : [after(1.5,sec) && r_aux==1 && r_error ==0]
  State_feat_ok -> state_update : [r_aux==1]
  data: i_enable input; i_desiredTest input; o_TestResult output; o_testDone output; r_aux local; i_motorStatus input; o_gear output; o_keyfob output; o_keyfobcom output; o_startButtom output; i_odometer input; i_speedmeter input; r_error local; r_odometer local; r_speedmeter local

== stateflow chart simulationSprint2/Chart ==
  state state_infinityLoop
    entry:
    if (i_keyfobValue==1)
    o_s1 = 1.5 ;
    o_s2 = 1.5 ;
    o_s3 = 1.2;
    elseif(i_keyfobValue==2)
    o_s1 = 5 ;
    o_s2 = 5;
    o_s3 = 5;
    else
    o_s1 = 11 ;
    o_s2 = 11 ;
    o_s3 = 11;
    end
  (default) -> state_infinityLoop
  state_infinityLoop -> state_infinityLoop : after(100,msec)
  data: i_keyfobValue input; o_s1 output; o_s2 output; o_s3 output

== stateflow chart simulationSprint2/SelectTest ==
  state state_idle
    entry:
    r_aux=0;
    o_testResult = 0 ;
    o_enable = 0;
  state state_SendRequestTest
    during:
    o_req=(i_req);
    on after(100,msec):
    o_enable = 1;
    exit:
    o_enable = 0;
  state state_WaitTest
    during :
  state state_update
    entry:
    r_aux = 0;
    o_testResult = i_testResult;
    o_testEnd = 1;
    on after(100,msec):
    r_aux=1;
  state state_pause
    during :
    o_testEnd  = 0 ;
  (default) -> state_idle
  state_idle -> state_SendRequestTest : [i_enable==1]
  state_SendRequestTest -> state_WaitTest : [o_enable==1]
  state_WaitTest -> state_update : [i_done==1]
  state_update -> state_pause : [r_aux==1]
  data: i_req input; i_enable input int8; o_req output int8; o_enable output int8; i_done input int8; i_testResult input int8; o_testResult output int8; r_aux local; o_testEnd output

== stateflow chart simulationSprint2/Chart1 ==
  note: The module responsible by send the correct dds value to module.
      |
      | Notice : i_ means input signals
      | 		o_ means output signals
      |
      | Input :
      | i_ddsCommand - DDS commands. 1- Unfold the mirrors ; 0- Fold the mirrors
      | i_LockCommand - Lock commands. 1 - Lock the doors - 0 - unlock the doors
      | Output :
      | o_ddsCommand - Value dds to the system module.
  state state_selectDataOutput
    entry:
    o_ddsCommand =0;
    during :
    if (i_ddsCommand==0)
    o_ddsCommand = 2;
    elseif(i_ddsCommand==1)
    o_ddsCommand = 3;
    elseif(i_LockCommand==1)
    o_ddsCommand = 4;
    elseif(i_LockCommand==0)
    o_ddsCommand = 5;
    end
  (default) -> state_selectDataOutput
  data: i_ddsCommand input; i_LockCommand input; o_ddsCommand output

== stateflow chart simulationSprint2/SyncWelcomeFeature "Req 11" ==
  note: The module responsible by test the requeriment eleven.
      |
      | Notice : i_ means input signals
      | 		o_ means output signals
      |
      | Input :
      | i_enable - Start the test. 1- Start test . 0 - Do nothing.
      | i_desiredTest - Test Number Value. All the modules recieve the
      | signal and decide either execute the test. Ex: Value "1" means that will being testing the requeriment 1.
      | i_Sync. 0 - Showing nothing ; 1 - Showing Welcome ; 2 - Radio Mode.
      |
      |
      | Output :
      | o_TestResult - Result of test. 1 - Test ran correctly ; 2 - Test ran incorrectly.
      | o_TestDone - Test has been completed. 1 - Completed ;
      | o_keyfob - Signal that indicates if the key is inside or not from the car. 1 - Key inside ; 0 - Key outside.
      | o_keyCommand - Signal to lock or unlock the car. "1 - lock the car ; 0 - Unlock the car" ;  -1 - Do nothing.
      | o_openTheDoor - Signal to represent the opening the door. 1 - Opening ; 0 - Closing ; -1 - Do nothing.
  state State_idle
    entry :
    r_aux=0;
    o_TestResult = 0;
    o_KeyfobCommand =0;
    r_error = 0;
    during:
  state state_checkSync
    entry:
    r_aux =0;
    o_openTheDoor =1;
    during:
    on after(200,msec):
    if(i_Sync~=1)
    r_error = 1;
    end
    on after(1,sec):
    o_openTheDoor =0;
    exit:
    r_aux=0;
  state state_readyingSystem
    during:
    o_openTheDoor =0;
    on after(200,msec):
    r_aux=1;
    exit : r_aux=0;
  state state_testRadio
    during :
    on after(400,msec):
    r_aux=1;
    exit :
    r_aux=0;
  state State_error
    during:
    o_TestResult =0;
    o_testDone =1 ;
    on after(500,msec):
    r_aux =1;
    exit :
    r_aux =0;
  state State_feat_ok
    during:
    o_TestResult =1;
    o_testDone =1;
    on after(100,msec):
    r_aux =1;
    exit:
    r_aux =0;
  state state_update
    entry:
    r_aux = 0;
    on after(500,msec):
    during:
    o_TestResult =0;
    o_testDone = 0;
    r_aux =1 ;
    exit:
  (default) -> State_idle
  State_idle -> state_readyingSystem : [i_enable==1 && i_desiredTest ==11 ]
  state_readyingSystem -> state_checkSync : [r_aux==1]
  state_checkSync -> State_error [order 2] : [after(5,sec) &&  r_error == 1]
  state_update -> State_idle : [r_aux==1]
  state_checkSync -> state_testRadio [order 1] : [after(5,sec) && r_error == 0]
  state_testRadio -> State_error [order 2] : [i_Sync~=2 && r_aux==1]
  state_testRadio -> State_feat_ok [order 1] : [i_Sync==2 && r_aux ==1]
  State_error -> state_update : [r_aux==1]
  State_feat_ok -> state_update : [r_aux==1]
  data: o_TestResult output; r_aux local; i_desiredTest input; i_enable input; i_Sync input; r_error local; o_testDone output; o_openTheDoor output int8; o_KeyfobCommand output

== stateflow chart simulationSprint2/"Req 1" ==
  note: The module responsible by test the requeriment one.
      |
      | Notice : i_ means input signals
      | 		o_ means output signals
      |
      | Input :
      | i_enable = Start the test. 1- Start test . 0 - Do nothing.
      | i_desiredTest = Test Number Value. All the modules recieve the
      | signal and decide either execute the test. Ex: Value "1" means that will being testing the requeriment 1.
      | i_WindowRightState = Windows State. 1- Windows Opening  ; 0 - Windows Closing ;  -1 - Do nothing.
      | i_WindowLeftState = Windows State. 1- Windows Opening  ; 0 - Windows Closing ;  -1 - Do nothing.
      | Output :
      | o_keyfob = Signal to lock or unlock the car. 1 - lock the car ; 0 - Unlock the car ;  -1 - Do nothing.
      | o_CloseDoor = Signal to generate the open or close door. 1 - Open Door ; 0 - Close Door.
      | o_TestResult = Result of test. 1 - Test ran correctly ; 2 - Test ran incorrectly.
      | o_TestDone = Test has been completed. 1- Completed ;
  state State_idle
    entry :
    r_aux=0;
    r_count = 1 ;
    o_TestResult = -1;
    r_error = 0;
    o_CloseDoor = 0 ;
    during:
  state state_readyingSystem
    entry :
    during:
    o_keyfobCom =2;
    on after(0.2,sec):
    o_keyfobCom =0;
    o_CloseDoor =0;
    on after(0.8,sec):
    o_keyfobCom =1;
    on after(1.2,sec):
    o_keyfobCom =0;
    on after(1.5,sec):
    r_aux=1;
    exit : r_aux=0;
  state State_feat_ok
    during:
    o_TestResult =1;
    o_testDone =1;
    on after(100,msec):
    r_aux =1;
    exit:
    r_aux =0;
  state State_error
    during:
    o_TestResult =0;
    o_testDone =1 ;
    on after(100,msec):
    r_aux =1;
    exit :
    r_aux =0;
  state state_update
    entry:
    r_aux = 0;
    on after(200,msec):
    during:
    o_keyfobCom = -1;
    o_TestResult =-1;
    o_testDone = 0;
    r_aux =1 ;
    exit:
  (default) -> State_idle
  State_idle -> state_readyingSystem : [i_enable==1 && i_desiredTest ==1 ]
  state_readyingSystem -> State_feat_ok [order 1] : [r_aux==1 && i_WindowRightState==1 && i_WindowLeftState==1]
  state_update -> State_idle : [r_aux==1]
  state_readyingSystem -> State_error [order 2] : [r_aux==1 && (i_WindowRightState~=1 && i_WindowLeftState~=1)]
  State_feat_ok -> state_update : [r_aux==1]
  State_error -> state_update : [r_aux==1]
  data: o_TestResult output; r_aux local; i_desiredTest input; i_enable input; i_WindowRightState input; r_error local; o_testDone output; r_count local; o_CloseDoor output; i_WindowLeftState input; o_keyfobCom output

== stateflow chart simulationSprint2/Req3 ==
  note: The module responsible by test the requeriment three.
      |
      | Notice : i_ means input signals
      | 		o_ means output signals
      |
      | Input :
      | i_enable - Start the test. 1- Start test . 0 - Do nothing.
      | i_desiredTest - Test Number Value. All the modules recieve the
      | signal and decide either execute the test. Ex: Value "1" means that will being testing the requeriment 1.
      | i_mirrorLeft - Fold or Unfold mirror state . 1 - Mirror is unfold.  0 - Mirror is fold.
      | i_mirrorRight - Fold or Unfold mirror state . 1 - Mirror is unfold.  0 - Mirror is fold.
      | i_LeftDoorBackLockState. State of the door. 1 - Unlock ;  0 - Lock .
      | i_RightDoorBackLockState. State of the door. 1 - Unlock ;  0 - Lock .
      | i_LeftWindowBackState . 1- Windows Opening  ; 0 - Windows Closing ;  -1 - Do nothing.
      | i_RightWindowBackState . 1- Windows Opening  ; 0 - Windows Closing ;  -1 - Do nothing.
      |
      | Output :
      | o_TestResult - Result of test. 1 - Test ran correctly ; 2 - Test ran incorrectly.
      | o_TestDone - Test has been completed. 1 - Completed ;
      | o_keyfob - Signal that indicates if the key is inside or not from the car. 1 - Key inside ; 0 - Key outside.
      | o_keyfobCommand - Signal to lock or unlock the car. "1 - lock the car ; 0 - Unlock the car" ;  -1 - Do nothing.
      | o_ddsCommand - 3 - Unfold Mirror ; 2 - Fold Mirror.
      | o_startButtom - Signal to start or off the car. 1- Car Start ; 0 - Car off.
      | o_gear = gear State ; 1 - Park ; 0 - Engaged.
  state state_mirror_dds_unfold
    during:
    o_keyfobCommand = 0;
    on after(100,msec):
    o_keyfob = 1;
    on after(200,msec):
    o_gear = 1;
    on after(300,msec):
    o_startButtom =1;
    on after(1.3,sec):
    o_ddsCommand =2;
    on after(5,sec):
    r_aux=1;
    exit:
    r_aux = 0 ;
  state state_unlockCar
    during:
    o_keyfobCommand = 2;
    on after(100,msec):
    o_keyfobCommand = 0;
    o_keyfob = 1;
    on after(200,msec):
    o_ddsCommand = 0;
    on after(1,sec):
    r_aux=1;
    exit:
    r_aux = 0
  state state_mirror_fold_lock
    during:
    on after(100,msec):
    o_keyfobCommand = 1 ;
    o_ddsCommand = 0 ;
    on after(150,msec):
    o_keyfobCommand = 0;
    on after(200,msec):
    o_keyfob = 0;
    on after(3,sec):
    r_aux=1;
    exit:
    r_aux = 0 ;
  state state_idle
    entry :
    r_aux = 0 ;
    o_ddsCommand = 0 ;
    o_keyfobCommand = 0 ;
    o_startButtom = 0 ;
    o_gear = 1;
  state State_error
    during:
    o_TestResult =0;
    o_testDone =1 ;
    on after(100,msec):
    r_aux =1;
    exit :
    r_aux =0;
  state stateWithCarOn
    during :
    o_ddsCommand =3;
    on after(3,sec):
    r_aux=1;
    exit:
    r_aux = 0 ;
  state stateWithCarOff
    during :
    o_ddsCommand =7;
  state State_feat_ok
    during:
    o_TestResult =1;
    o_testDone =1;
    on after(100,msec):
    r_aux =1;
    exit:
    r_aux =0;
  state state_update
    entry:
    r_aux = 0;
    on after(100,msec):
    o_testDone = 0;
    during:
    o_TestResult =0;
  state_mirror_fold_lock -> state_unlockCar [order 2] : [r_aux==1 && i_mirrorRight == 0 && i_mirrorLeft == 0 ]
  state_unlockCar -> state_mirror_dds_unfold [order 1] : [r_aux==1 && i_mirrorRight ==1 && i_mirrorLeft == 1 ]
  (default) -> state_idle
  state_idle -> state_mirror_fold_lock : [i_enable ==1 && i_desiredTest == 3]
  state_mirror_dds_unfold -> State_error [order 2] : [r_aux==1 && i_mirrorRight ==1 && i_mirrorLeft == 1 ]
  state_update -> state_idle : [after(200,msec)]
  state_mirror_dds_unfold -> stateWithCarOn [order 1] : [r_aux==1 && i_mirrorRight ==0 && i_mirrorLeft == 0 ]
  state_unlockCar -> State_error [order 2] : [r_aux==1 && i_mirrorRight ==0 && i_mirrorLeft == 0 ]
  state_mirror_fold_lock -> State_error [order 1] : [r_aux==1 && i_mirrorRight ~= 0 && i_mirrorLeft ~= 0 ]
  stateWithCarOn -> State_error [order 1] : [r_aux==1 && i_mirrorRight ==0 && i_mirrorLeft == 0 ]
  State_error -> state_update : [r_aux==1]
  stateWithCarOff -> State_error [order 1] : [after(3,sec) && ( i_RightDoorBackLockState ~= 1 || i_LeftDoorBackLockState ~= 1 || i_RightWindowBackState ~= 1 || i_LeftWindowBackState ~= 1) ]
  stateWithCarOn -> stateWithCarOff [order 2] : [r_aux==1 && i_mirrorRight ==1 && i_mirrorLeft == 1 ]
  stateWithCarOff -> State_feat_ok [order 2] : [after(3,sec) && i_RightDoorBackLockState == 1 && i_LeftDoorBackLockState == 1  && i_RightWindowBackState == 1 && i_LeftWindowBackState == 1]
  State_feat_ok -> state_update : [r_aux==1]
  data: i_enable input; i_desiredTest input; o_TestResult output; o_testDone output; r_aux local; i_mirrorLeft input; o_keyfob output; o_ddsCommand output; o_keyfobCommand output; i_mirrorRight input; o_startButtom output; o_gear output; i_LeftDoorBackLockState input; i_RightDoorBackLockState input; i_LeftWindowBackState input; i_RightWindowBackState input
